simulink model "IDEAL_Diagrama_completo_prolijo"  (R2023b)
settings: Solver=VariableStepAuto  StartTime=0.0  StopTime=15  FixedStep=Ts  RelTol=1e-3
values from neighbouring files (symbols this model uses):
  A_corriente = [0 1; -wn_corriente^2 -2*zeta_corriente*wn_corriente]    [SensoresReales.m]
  A_inv = [0 1; -wn_inv^2 -2*zeta_inv*wn_inv]    [SensoresReales.m]
  A_temp = -1/tau_temp    (= -0.05)    [SensoresReales.m]
  A_tita = [0 1; -wn_tita^2 -2*zeta_tita*wn_tita]    [SensoresReales.m]
  B_corriente = [0; wn_corriente^2]    [SensoresReales.m]
  B_inv = [0; wn_inv^2]    [SensoresReales.m]
  B_temp = 1/tau_temp    (= 0.05)    [SensoresReales.m]
  B_tita = [0; wn_tita^2]    [SensoresReales.m]
  ba = Jeq * n * wn    [PolosPID.m]
  C_corriente = [1 0]    [SensoresReales.m]
  C_inv = [1 0]    [SensoresReales.m]
  C_temp = 1    [SensoresReales.m]
  C_tita = [1 0]    [SensoresReales.m]
  D_corriente = 0    [SensoresReales.m]
  D_inv = 0    [SensoresReales.m]
  D_temp = 0    [SensoresReales.m]
  D_tita = 0    [SensoresReales.m]
  ketita = double(sol.ketita_s)    [PIDPolosObsReducidoEst.m]    (also in PolosObsReducidoEst.m)
  kew = double(sol.kew_s)    [PIDPolosObsReducidoEst.m]    (also in PolosObsReducidoEst.m)
  kewint = double(sol.kewint_s)    [PIDPolosObsReducidoEst.m]    (also in PolosObsReducidoEst.m = 0)
  Ksa = Jeq * n * wn^2    [PolosPID.m]
  Ksia = Jeq * wn^3    [PolosPID.m]
  Ra_prima = Lq/Tau    [RaLazoControlCorriente.m]
  Tau = -1/Pi    (= 0.0002)    [RaLazoControlCorriente.m]
  Ts = 0.0001    [TustinPID.m]
undefined symbols (not defined in the file or in its folder): alfa, beq, Cts, dGi, dGsc, dGsp, dGsT, femax, g, gcbh, id0, io0, iq0, Ismax, Isnom, Jeq, KEeq, kl, KTeq, lambda_m, Ld, Lls, Lq, nGi, nGsc, nGsp, nGsT, Pp, r, Rs, Rts_amb, sps, sps_rtmsupport, tita0, Tqnom, Ts0, Tsmax, Vflnom, Vsat, Wlnom, wm0, Wmnom
libraries: simulink_extras x8, eeTransforms x4, simulink x4, SignalEditorBlockLib x3, spsPositiveSequencePLLDrivenLib x1, spsSecondOrderFilterLib x1, spsMeanVariableFrequencyLib x1, spsabctodq0Lib x1
settings Model: Creator=Julian  LastModifiedBy=Gustavo

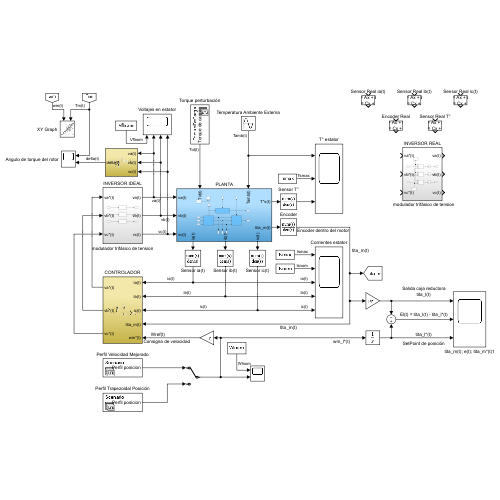
[thumbnail: Simulink's stored preview of the top-level diagram]
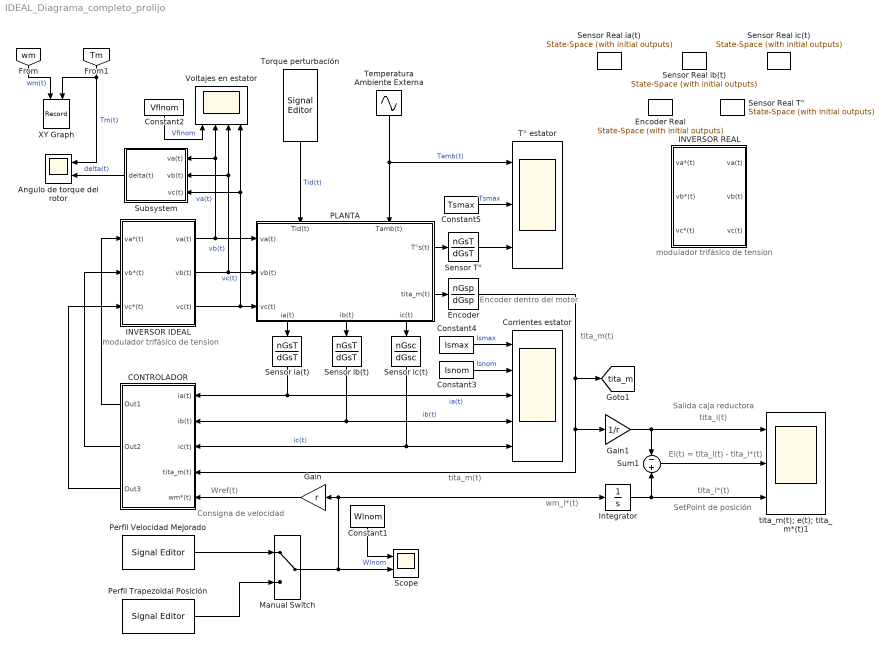
== system IDEAL_Diagrama_completo_prolijo ==
  note: modulador trifásico de tension
  note: SetPoint de posición
  note: Wref(t)
  note: Salida caja reductora
  note: Encoder dentro del motor
  note: tita_m(t)
  note: El(t) = tita_l(t) - tita_l*(t)
  note: tita_l*(t)
  note: tita_m(t)
  note: wm_l*(t)
  note: tita_l(t)
  note: Consigna de velocidad
  note: modulador trifásico de tension
  Angulo de torque del rotor : Scope  NumInputPorts=2
  CONTROLADOR : Subsystem
  Constant1 : Constant  Value=Wlnom
  Constant2 : Constant  Value=Vflnom
  Constant3 : Constant  Value=Isnom
  Constant4 : Constant  Value=Ismax
  Constant5 : Constant  Value=Tsmax
  Corrientes estator : Scope  NumInputPorts=5
  Encoder : TransferFcn  Numerator=nGsp  Denominator=dGsp
  Encoder Real : simulink_extras/Additional Linear/State-Space (with initial outputs)  A=A_tita  B=B_tita  C=C_tita  D=D_tita  U0=0  Y0=0
  Gain : Gain  Gain=r
  Gain1 : Gain  Gain=1/r
  INVERSOR IDEAL : Subsystem
  INVERSOR REAL : Subsystem
  Integrator : Integrator
  Manual Switch : ManualSwitch
  PLANTA : Subsystem
      settings: PortSchema="{\"entries\":[{\"content\":{\"sides\":[{\"content\":{\"connectorIds\":[\"In1\",\"In2\",\"In3\"]},\"type\":\"ConnectorPlacement.EquallySpacedRectSide\",\"uuid\":\"c9ff8e03-575d-49b6-9d53-263c6173ec7a\"},{\"content\":{\"connectorIds\":[\"Out1\",\"Out2\"],\"side\":\"RIGHT\"},\"type\":\"ConnectorPlacement.EquallySpacedRectSide\",\"uuid\":\"b812656a-111e-4032-91bd-eba1e3276cdf\"},{\"content\":{\"connectorIds\":[\"In4\",\"In5\"],\"side\":\"TOP\"},\"type\":\"ConnectorPlacement.EquallySpacedRectSide\",\"uuid\":\"1a03caaa-7f6e-4ad3-ab54-ee47607f786a\"},{\"content\":{\"connectorIds\":[\"Out3\",\"Out4\",\"Out5\"],\"side\":\"BOTTOM\"},\"type\":\"ConnectorPlacement.EquallySpacedRectSide\",\"uuid\":\"9d23a867-d392-4f38-a76b-2655c4618fc4\"}]},\"type\":\"ConnectorPlacement.EquallySpacedConnector\",\"uuid\":\"9323b1ce-1fa4-461e-b8aa-3e94b35b1dab\"}],\"packageUris\":[\"http://schema.mathworks.com/mf0/Connector/R2020b\"],\"version\":\"1.0\"}"
  Perfil Trapezoidal Posición : SignalEditorBlockLib/Signal Editor  FileName=Perfil trapezoidal de posicion.mat  ActiveScenario=Scenario  ActiveSignal=Perfil posicion  IsBus=off  OutputBusObjectStr=Bus: BusObject  SampleTime=0  ZeroCross=off  OutputAfterFinalValue=Setting to zero  Unit=inherit  PreserveSignalName=on  ApplySigPropsToAllScenarios=on  ApplySigPropsToAllSignals=off
  Perfil Velocidad Mejorado : SignalEditorBlockLib/Signal Editor  FileName=PerfilTrapezoidalVelocidadMejorado.mat  ActiveScenario=Scenario  ActiveSignal=Perfil posicion  IsBus=off  OutputBusObjectStr=Bus: BusObject  SampleTime=0  ZeroCross=off  OutputAfterFinalValue=Setting to zero  Unit=inherit  PreserveSignalName=on  ApplySigPropsToAllScenarios=on  ApplySigPropsToAllSignals=off
  Scope : Scope  NumInputPorts=2
  Sensor Real T° : simulink_extras/Additional Linear/State-Space (with initial outputs)  A=A_temp  B=B_temp  C=C_temp  D=D_temp  U0=Ts0  Y0=Ts0
  Sensor Real ia(t) : simulink_extras/Additional Linear/State-Space (with initial outputs)  A=A_corriente  B=B_corriente  C=C_corriente  D=D_corriente  U0=0  Y0=0
  Sensor Real ib(t) : simulink_extras/Additional Linear/State-Space (with initial outputs)  A=A_corriente  B=B_corriente  C=C_corriente  D=D_corriente  U0=0  Y0=0
  Sensor Real ic(t) : simulink_extras/Additional Linear/State-Space (with initial outputs)  A=A_corriente  B=B_corriente  C=C_corriente  D=D_corriente  U0=0  Y0=0
  Sensor T° : TransferFcn  Numerator=nGsT  Denominator=dGsT
  Sensor ia(t) : TransferFcn  Numerator=nGsT  Denominator=dGsT
  Sensor ib(t) : TransferFcn  Numerator=nGsT  Denominator=dGsT
  Sensor ic(t) : TransferFcn  Numerator=nGsc  Denominator=dGsc
  Subsystem : Subsystem
  Sum1 : Sum  Inputs=-|+
  Temperatura Ambiente Externa : Sin  Amplitude=27.5  Bias=12.5  Frequency=2*pi/15  Phase=pi/2  SampleTime=0
  Torque perturbación : SignalEditorBlockLib/Signal Editor  FileName=Torque de carga Tdl(t).mat  ActiveScenario=TorqueDeCarga  ActiveSignal=Torque de carga  IsBus=off  OutputBusObjectStr=Bus: BusObject  SampleTime=0  ZeroCross=off  OutputAfterFinalValue=Setting to zero  Unit=N*m  PreserveSignalName=on  ApplySigPropsToAllScenarios=on  ApplySigPropsToAllSignals=off
  T° estator : Scope  NumInputPorts=3
  Voltajes en estator : Scope  NumInputPorts=4
  XY Graph : Record  FileSettingsInternal="{\"entries\":[{\"content\":{\"excelSettings\":{\"content\":{},\"type\":\"Streamout.ExcelSettings\"}},\"type\":\"Streamout.FileSettingStorage\",\"uuid\":\"\"}],\"packageUris\":[\"http:\\/\\/schema.mathworks.com\\/mf0\\/streamout_blocks\\/R2020a\"],\"version\":\"1.0\"}"  Layout=[1 1]  SignalsInternal="{\"entries\":[{\"content\":{\"signals\":[{\"content\":{\"blockPath\":[],\"dimensions\":[1],\"domain\":\"\",\"lineColor\":\"#a2142f\",\"plots\":[1],\"port\":1,\"sid\":[\"\"],\"signalID\":587,\"signalName\":\"wm(t)\"},\"type\":\"RecordBlkView.Signal\",\"uuid\":\"\"},{\"content\":{\"blockPath\":[],\"dimensions\":[1],\"domain\":\"\",\"lineColor\":\"#139fff\",\"plots\":[1],\"port\":2,\"sid\":[\"\"],\"signalID\":591,\"signalName\":\"Tm(t)\"},\"type\":\"RecordBlkView.Signal\",\"uuid\":\"\"}]},\"type\":\"RecordBlkView.InputSignals\",\"uuid\":\"\"}],\"packageUris\":[\"http:\\/\\/schema.mathworks.com\\/mf0\\/streamout_blocks\\/R2020a\"],\"version\":\"1.0\"}"  VisualizationBindings="{\"xyplotplugin\":{\"info\":[{\"series\":[{\"bindingParametersList\":[{\"parameter\":\"Y-Axis\",\"signalID\":591,\"signalName\":\"Tm(t)\"},{\"parameter\":\"X-Axis\",\"signalID\":587,\"signalName\":\"wm(t)\"}],\"seriesID\":55069}],\"subplotID\":1}]}}"  CompatibilityTag=XY
  tita_m(t); e(t); tita_m*(t)1 : Scope  NumInputPorts=3
  tag scope: tita_m=global
  wires:
  INVERSOR IDEAL/1(va(t)) -> PLANTA/1(va(t)), Voltajes en estator/2, Subsystem/1(va(t))  "va(t)"
  INVERSOR IDEAL/2(vb(t)) -> PLANTA/2(vb(t)), Voltajes en estator/3, Subsystem/2(vb(t))  "vb(t)"
  INVERSOR IDEAL/3(vc(t)) -> Voltajes en estator/4, Subsystem/3(vc(t)), PLANTA/3(vc(t))  "vc(t)"
  CONTROLADOR/1(Out1) -> INVERSOR IDEAL/1(va*(t))
  CONTROLADOR/2(Out2) -> INVERSOR IDEAL/2(vb*(t))
  CONTROLADOR/3(Out3) -> INVERSOR IDEAL/3(vc*(t))
  Sensor T°/1 -> T° estator/3
  Gain/1 -> CONTROLADOR/5(wm*(t))
  Encoder/1 -> CONTROLADOR/4(tita_m(t)), Gain1/1, [tita_m]
  Gain1/1 -> tita_m(t); e(t); tita_m*(t)1/1, Sum1/1
  Sum1/1 -> tita_m(t); e(t); tita_m*(t)1/2
  Integrator/1 -> Sum1/2, tita_m(t); e(t); tita_m*(t)1/3
  PLANTA/3(ia(t)) -> Sensor ia(t)/1
  PLANTA/4(ib(t)) -> Sensor ib(t)/1
  PLANTA/5(ic(t)) -> Sensor ic(t)/1
  Temperatura Ambiente Externa/1 -> PLANTA/5(Tamb(t)), T° estator/1  "Tamb(t)"
  Torque perturbación/1 -> PLANTA/4(Tid(t))  "Tid(t)"
  PLANTA/2(tita_m(t)) -> Encoder/1
  PLANTA/1(T°s(t)) -> Sensor T°/1
  Sensor ic(t)/1 -> CONTROLADOR/3(ic(t)), Corrientes estator/5  "ic(t)"
  Sensor ib(t)/1 -> CONTROLADOR/2(ib(t)), Corrientes estator/4  "ib(t)"
  Sensor ia(t)/1 -> CONTROLADOR/1(ia(t)), Corrientes estator/3  "ia(t)"
  Manual Switch/1 -> Scope/2, Integrator/1, Gain/1
  Perfil Trapezoidal Posición/1 -> Manual Switch/2
  Perfil Velocidad Mejorado/1 -> Manual Switch/1
  Constant1/1 -> Scope/1  "Wlnom"
  Constant2/1 -> Voltajes en estator/1  "Vflnom"
  Constant3/1 -> Corrientes estator/2  "Isnom"
  Constant4/1 -> Corrientes estator/1  "Ismax"
  Subsystem/1(delta(t)) -> Angulo de torque del rotor/2  "delta(t)"
  [Tm] -> Angulo de torque del rotor/1, XY Graph/2  "Tm(t)"
  [wm] -> XY Graph/1  "wm(t)"
  Constant5/1 -> T° estator/2  "Tsmax"

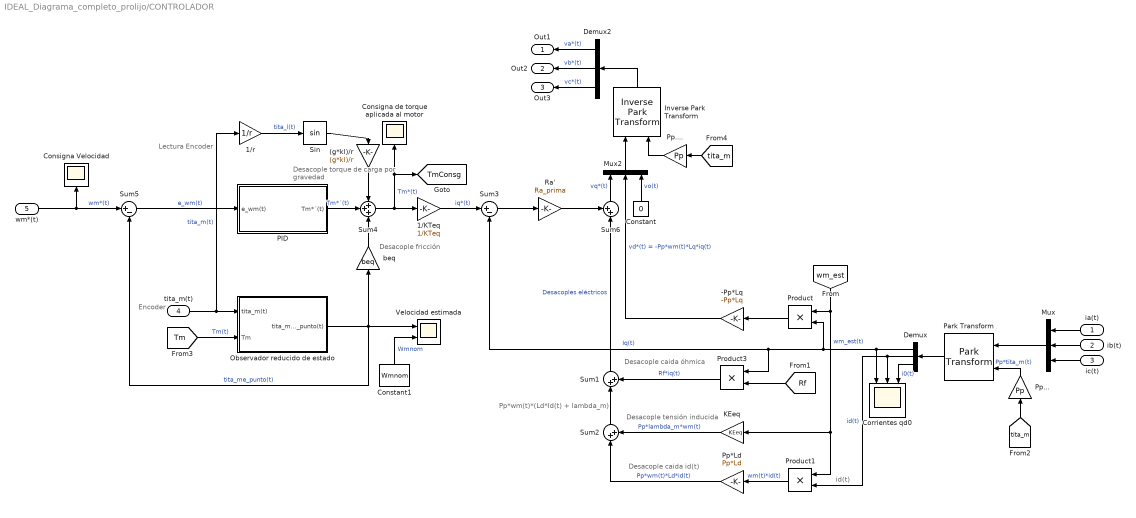
== system IDEAL_Diagrama_completo_prolijo/CONTROLADOR ==
  note: id(t)
  note: Desacople caida id(t)
  note: Encoder
  note: Desacople caida óhmica
  note: Desacople fricción
  note: Desacople tensión inducida
  note: Pp*wm(t)*(Ld*Id(t) + lambda_m)
  note: Lectura Encoder
  note: Desacople torque
      | de carga por gravedad
  ia(t) : Inport
  ib(t) : Inport  Port=2
  ic(t) : Inport  Port=3
  tita_m(t) : Inport  Port=4
  wm*(t) : Inport  Port=5
  (g*kl)/r : Gain  Gain=(g*kl)/r
  -Pp*Lq : Gain  Gain=-Pp*Lq
  1/KTeq : Gain  Gain=1/KTeq
  1/r : Gain  Gain=1/r
  Consigna Velocidad : Scope
  Consigna de torque aplicada al motor : Scope
  Constant : Constant  Value=0
  Constant1 : Constant  Value=Wmnom
  Corrientes qd0 : Scope  NumInputPorts=3
  Demux : Demux  Outputs=3
  Demux2 : Demux  Outputs=3
  Inverse Park Transform : eeTransforms/Inverse Park Transform  AxisAlignment=Q-axis  PowerInvariant=off
      settings: LibrarySourceBlock=|
      | ee_sl_lib/Mathematical
      | Transforms/Inverse
      | Park Transform
  KEeq : Gain  Gain=KEeq
  Mux : Mux  Inputs=3
  Mux2 : Mux  Inputs=3
  Observador reducido de estado : Subsystem
  PID : Subsystem
  Park Transform : eeTransforms/Park Transform  AxisAlignment=Q-axis  PowerInvariant=off
      settings: LibrarySourceBlock=|
      | ee_sl_lib/Mathematical
      | Transforms/Park Transform
  Pp*Ld : Gain  Gain=Pp*Ld
  Pp... : Gain  Gain=Pp
  Pp.... : Gain  Gain=Pp
  Product : Product
  Product1 : Product
  Product3 : Product
  Ra' : Gain  Gain=Ra_prima
  Sin : Trigonometry
  Sum1 : Sum  Inputs=|++
  Sum2 : Sum  Inputs=|++
  Sum3 : Sum  Inputs=|+-
  Sum4 : Sum  Inputs=+++
  Sum5 : Sum  Inputs=|+-
  Sum6 : Sum  Inputs=++|
  Velocidad estimada : Scope  NumInputPorts=2
  beq : Gain  Gain=beq
  Out1 : Outport
  Out2 : Outport  Port=2
  Out3 : Outport  Port=3
  tag scope: TmConsg=global
  wires:
  Mux/1 -> Park Transform/1
  [tita_m] -> Pp..../1
  Pp..../1 -> Inverse Park Transform/2
  Demux2/2 -> Out2/1  "vb*(t)"
  Sum3/1 -> Ra'/1
  Constant/1 -> Mux2/3  "vo(t)"
  Demux2/1 -> Out1/1  "va*(t)"
  -Pp*Lq/1 -> Mux2/2  "vd*(t) = -Pp*wm(t)*Lq*iq(t)"
  Product3/1 -> Sum1/2  "Rf*iq(t)"
  [tita_m] -> Pp.../1
  Ra'/1 -> Sum6/1
  Inverse Park Transform/1 -> Demux2/1
  KEeq/1 -> Sum2/2  "Pp*lambda_m*wm(t)"
  Product1/1 -> Pp*Ld/1  "wm(t)*id(t)"
  Mux2/1 -> Inverse Park Transform/1
  Sum2/1 -> Sum1/1
  wm*(t)/1 -> Sum5/1, Consigna Velocidad/1  "wm*(t)"
  Pp*Ld/1 -> Sum2/1  "Pp*wm(t)*Ld*id(t)"
  1/KTeq/1 -> Sum3/1  "iq*(t)"
  Product/1 -> -Pp*Lq/1
  ia(t)/1 -> Mux/1
  Park Transform/1 -> Demux/1
  Pp.../1 -> Park Transform/2  "Pp*tita_m(t)"
  Sum6/1 -> Mux2/1  "vq*(t)"
  Demux2/3 -> Out3/1  "vc*(t)"
  ib(t)/1 -> Mux/2
  tita_m(t)/1 -> 1/r/1, Observador reducido de estado/1(tita_m(t))  "tita_m(t)"
  [Tm] -> Observador reducido de estado/2(Tm)  "Tm(t)"
  [Rf] -> Product3/2
  ic(t)/1 -> Mux/3
  Sum5/1 -> PID/1(e_wm(t))  "e_wm(t)"
  Sum1/1 -> Sum6/2  "Desacoples eléctricos"
  PID/1(Tm*´(t)) -> Sum4/2  "Tm*´(t)"
  Sum4/1 -> 1/KTeq/1, Consigna de torque aplicada al motor/1, [TmConsg]  "Tm*(t)"
  beq/1 -> Sum4/3
  Observador reducido de estado/1(tita_me_punto(t)) -> beq/1, Velocidad estimada/1, Sum5/2  "tita_me_punto(t)"
  Demux/3 -> Corrientes qd0/3  "i0(t)"
  Demux/2 -> Product1/2, Corrientes qd0/2  "id(t)"
  Demux/1 -> Product3/1, Sum3/2, Product/2, Corrientes qd0/1  "Iq(t)"
  1/r/1 -> Sin/1  "tita_l(t)"
  Sin/1 -> (g*kl)/r/1
  (g*kl)/r/1 -> Sum4/1
  [wm_est] -> Product/1, Product1/1, KEeq/1  "wm_est(t)"
  Constant1/1 -> Velocidad estimada/2  "Wmnom"

== system IDEAL_Diagrama_completo_prolijo/INVERSOR IDEAL ==
  va*(t) : Inport
  vb*(t) : Inport  Port=2
  vc*(t) : Inport  Port=3
  Inversor fase a : TransferFcn  Numerator=nGi  Denominator=dGi
  Inversor fase b : TransferFcn  Numerator=nGi  Denominator=dGi
  Inversor fase c : TransferFcn  Numerator=nGi  Denominator=dGi
  va(t) : Outport
  vb(t) : Outport  Port=2
  vc(t) : Outport  Port=3
  wires:
  Inversor fase c/1 -> vc(t)/1  "vc(t)"
  va*(t)/1 -> Inversor fase a/1
  Inversor fase a/1 -> va(t)/1  "va(t)"
  vc*(t)/1 -> Inversor fase c/1
  Inversor fase b/1 -> vb(t)/1  "vb(t)"
  vb*(t)/1 -> Inversor fase b/1

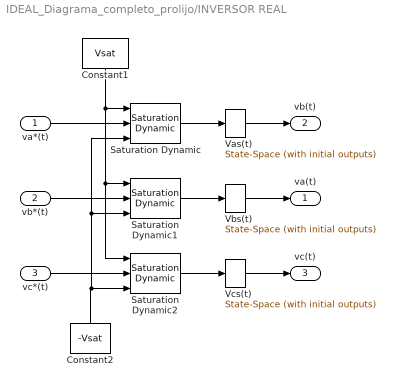
== system IDEAL_Diagrama_completo_prolijo/INVERSOR REAL ==
  va*(t) : Inport
  vb*(t) : Inport  Port=2
  vc*(t) : Inport  Port=3
  Constant1 : Constant  Value=Vsat
  Constant2 : Constant  Value=-Vsat
  Saturation Dynamic : simulink/Discontinuities/Saturation Dynamic  OutMin=[]  OutMax=[]  OutDataTypeStr=Inherit: Same as second input  OutDataType=fixdt(1, 16)  OutScaling=2^-10  DoSatur=off
  Saturation Dynamic1 : simulink/Discontinuities/Saturation Dynamic  OutMin=[]  OutMax=[]  OutDataTypeStr=Inherit: Same as second input  OutDataType=fixdt(1, 16)  OutScaling=2^-10  DoSatur=off
  Saturation Dynamic2 : simulink/Discontinuities/Saturation Dynamic  OutMin=[]  OutMax=[]  OutDataTypeStr=Inherit: Same as second input  OutDataType=fixdt(1, 16)  OutScaling=2^-10  DoSatur=off
  "Vas(t) " : simulink_extras/Additional Linear/State-Space (with initial outputs)  A=A_inv  B=B_inv  C=C_inv  D=D_inv  U0=0  Y0=0
  "Vbs(t) " : simulink_extras/Additional Linear/State-Space (with initial outputs)  A=A_inv  B=B_inv  C=C_inv  D=D_inv  U0=0  Y0=0
  "Vcs(t) " : simulink_extras/Additional Linear/State-Space (with initial outputs)  A=A_inv  B=B_inv  C=C_inv  D=D_inv  U0=0  Y0=0
  va(t) : Outport
  vb(t) : Outport  Port=2
  vc(t) : Outport  Port=3
  wires:
  va*(t)/1 -> Saturation Dynamic/2
  vb*(t)/1 -> Saturation Dynamic1/2
  vc*(t)/1 -> Saturation Dynamic2/2
  Constant2/1 -> Saturation Dynamic2/3, Saturation Dynamic/3, Saturation Dynamic1/3
  Saturation Dynamic/1 -> "Vas(t) "/1
  "Vas(t) "/1 -> vb(t)/1
  Saturation Dynamic1/1 -> "Vbs(t) "/1
  Saturation Dynamic2/1 -> "Vcs(t) "/1
  "Vbs(t) "/1 -> va(t)/1
  "Vcs(t) "/1 -> vc(t)/1
  Constant1/1 -> Saturation Dynamic2/1, Saturation Dynamic1/1, Saturation Dynamic/1

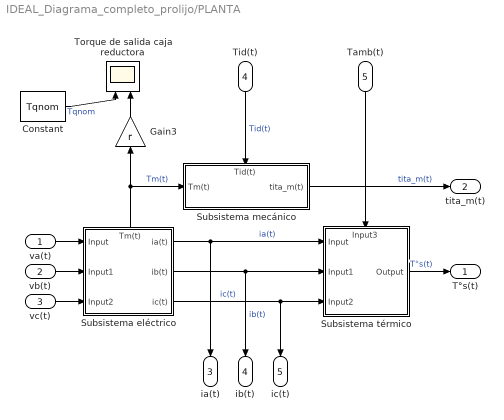
== system IDEAL_Diagrama_completo_prolijo/PLANTA ==
  va(t) : Inport
  vb(t) : Inport  Port=2
  vc(t) : Inport  Port=3
  Tid(t) : Inport  Port=4
  Tamb(t) : Inport  Port=5
  Constant : Constant  Value=Tqnom
  Gain3 : Gain  Gain=r
  Subsistema eléctrico : Subsystem
      settings: PortSchema="{\"entries\":[{\"content\":{\"sides\":[{\"content\":{\"connectorIds\":[\"In1\",\"In2\",\"In3\"]},\"type\":\"ConnectorPlacement.EquallySpacedRectSide\",\"uuid\":\"55314de5-b6ab-4161-b15d-819ac9b3d610\"},{\"content\":{\"connectorIds\":[\"Out1\",\"Out2\",\"Out3\"],\"side\":\"RIGHT\"},\"type\":\"ConnectorPlacement.EquallySpacedRectSide\",\"uuid\":\"6d89c228-26ff-4db5-b942-5bfef0be2fde\"},{\"content\":{\"connectorIds\":[\"Out4\"],\"side\":\"TOP\"},\"type\":\"ConnectorPlacement.EquallySpacedRectSide\",\"uuid\":\"a52f3ca3-a7f6-4886-b92b-9c9e6a107711\"}]},\"type\":\"ConnectorPlacement.EquallySpacedConnector\",\"uuid\":\"22991da4-d60d-4ddc-8bfe-b68e23663f11\"}],\"packageUris\":[\"http://schema.mathworks.com/mf0/Connector/R2020b\"],\"version\":\"1.0\"}"
  Subsistema mecánico : Subsystem
      settings: PortSchema="{\"entries\":[{\"content\":{\"sides\":[{\"content\":{\"connectorIds\":[\"In1\"]},\"type\":\"ConnectorPlacement.EquallySpacedRectSide\",\"uuid\":\"db0c31ff-fb9a-4cce-bd75-6b297d65744d\"},{\"content\":{\"connectorIds\":[\"Out1\"],\"side\":\"RIGHT\"},\"type\":\"ConnectorPlacement.EquallySpacedRectSide\",\"uuid\":\"ab44173d-bb84-4ea2-b7b7-ef15b1ff9d5e\"},{\"content\":{\"connectorIds\":[\"In2\"],\"side\":\"TOP\"},\"type\":\"ConnectorPlacement.EquallySpacedRectSide\",\"uuid\":\"a2ba5669-abba-4e87-b14b-37ec0d904023\"}]},\"type\":\"ConnectorPlacement.EquallySpacedConnector\",\"uuid\":\"7722c9ef-afaa-4930-9e2a-97c0dfb446ab\"}],\"packageUris\":[\"http://schema.mathworks.com/mf0/Connector/R2020b\"],\"version\":\"1.0\"}"
  Subsistema térmico : Subsystem
      settings: PortSchema="{\"entries\":[{\"content\":{\"sides\":[{\"content\":{\"connectorIds\":[\"In1\",\"In2\",\"In3\"]},\"type\":\"ConnectorPlacement.EquallySpacedRectSide\",\"uuid\":\"499bb5e3-da94-498d-be5e-1974ba0b4a58\"},{\"content\":{\"connectorIds\":[\"Out1\"],\"side\":\"RIGHT\"},\"type\":\"ConnectorPlacement.EquallySpacedRectSide\",\"uuid\":\"13ea5dea-e51e-4770-b579-88e3e6e50884\"},{\"content\":{\"connectorIds\":[\"In4\"],\"side\":\"TOP\"},\"type\":\"ConnectorPlacement.EquallySpacedRectSide\",\"uuid\":\"72517ed1-a98f-428e-86e2-c370e237c602\"}]},\"type\":\"ConnectorPlacement.EquallySpacedConnector\",\"uuid\":\"7e0eda24-12d6-49d0-ad1f-024c88e78140\"}],\"packageUris\":[\"http://schema.mathworks.com/mf0/Connector/R2020b\"],\"version\":\"1.0\"}"
  Torque de salida caja reductora : Scope  NumInputPorts=2
  T°s(t) : Outport
  tita_m(t) : Outport  Port=2
  ia(t) : Outport  Port=3
  ib(t) : Outport  Port=4
  ic(t) : Outport  Port=5
  wires:
  Tamb(t)/1 -> Subsistema térmico/4(Input3)
  Subsistema eléctrico/3(ic(t)) -> Subsistema térmico/3(Input2), ic(t)/1  "ic(t)"
  Subsistema eléctrico/1(ia(t)) -> Subsistema térmico/1(Input), ia(t)/1  "ia(t)"
  Subsistema térmico/1(Output) -> T°s(t)/1  "T°s(t)"
  Subsistema eléctrico/4(Tm(t)) -> Gain3/1, Subsistema mecánico/1(Tm(t))  "Tm(t)"
  Subsistema eléctrico/2(ib(t)) -> Subsistema térmico/2(Input1), ib(t)/1  "ib(t)"
  Subsistema mecánico/1(tita_m(t)) -> tita_m(t)/1  "tita_m(t)"
  va(t)/1 -> Subsistema eléctrico/1(Input)
  vb(t)/1 -> Subsistema eléctrico/2(Input1)
  Tid(t)/1 -> Subsistema mecánico/2(Tid(t))  "Tid(t)"
  vc(t)/1 -> Subsistema eléctrico/3(Input2)
  Gain3/1 -> Torque de salida caja reductora/2
  Constant/1 -> Torque de salida caja reductora/1  "Tqnom"

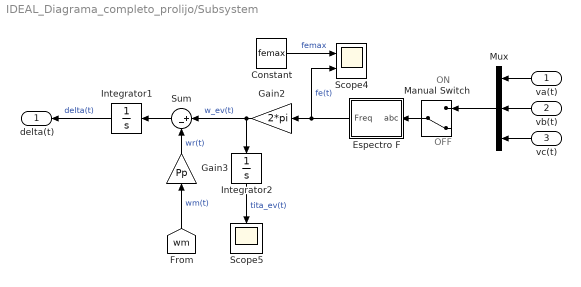
== system IDEAL_Diagrama_completo_prolijo/Subsystem ==
  note: OFF
  note: ON
  va(t) : Inport
  vb(t) : Inport  Port=2
  vc(t) : Inport  Port=3
  Constant : Constant  Value=femax
  Espectro F : Subsystem  AncestorBlock=|  DialogController=POWERSYS.PowerSysDialog  LoadFcn=sps_rtmsupport('LoadFcn', gcbh);  StartFcn=sps_rtmsupport('StartFcn', gcbh);  StopFcn=sps_rtmsupport('StopFcn', gcbh);  mask(PLL (3ph)){Fmin=45, Par_Init=[0, 50], ParK=[180, 3200, 1], TcD=1e-4, MaxRateChangeFreq=12, FilterCutOffFreq=25, Ts=0, AGC=on}
      | sps_lib/Control/PLL
      | (3ph)
      mask prompts: Fmin "Minimum frequency (Hz):"; Par_Init "Initial inputs [ Phase (degrees), Frequency (Hz) ]:"; ParK "Regulator gains [ Kp, Ki, Kd ]:"; TcD "Time constant for derivative action (s):"; MaxRateChangeFreq "Maximum rate of change of frequency (Hz/s):"; FilterCutOffFreq "Filter cut-off frequency for frequency measurement (Hz):"; Ts "Sample time:"; AGC "Enable automatic gain control"
      mask help:
      | This Phase Locked Loop (PLL) system can be used  to synchronize on a set of variable frequency, three-phase sinusoidal signals. If the Automatic Gain Control is enabled, the input (phase error) of the PLL regulator is scaled according to the input signals magnitude.
      |
      | For optimal performance, set regulator gains [ Kp Ki  Kd ] = [ 180  3200  1 ] and check the Enable Automatic Gain Control parameter.
      |
      | Input : Vector containing the normalized three-phase signals [Va Vb Vc]
      | Output 1:  Measured frequency (Hz) = w/(2pi)
      | Output 2:  Ramp w.t varying between  0 and 2*pi, synchronized on zero crossings of the fundamental (positive-sequence) of phase A.
      mask init:
      | block=gcb;
      | [WantBlockChoice,Ts,sps] = powericon('PLL3phInit',block,Fmin,Par_Init,ParK,TcD, MaxRateChangeFreq, FilterCutOffFreq, AGC,Ts);
      | powericon('SetInternalModels','set',block,WantBlockChoice);
      settings: CopyFcn=sps_rtmsupport('CopyFcn', gcbh);  DeleteFcn=sps_rtmsupport('DeleteFcn', gcbh);  UndoDeleteFcn=sps_rtmsupport('UndoDeleteFcn', gcbh);  ModelCloseFcn=sps_rtmsupport('ModelCloseFcn', gcbh);  PreSaveFcn=sps_rtmsupport('PreSaveFcn', gcbh);  PostSaveFcn=sps_rtmsupport('PostSaveFcn', gcbh);  NameChangeFcn=sps_rtmsupport('NameChangeFcn', gcbh);  PreCopyFcn=sps_rtmsupport('PreCopyFcn', gcbh);  OpenFcn=sps_rtmsupport('OpenFcn', gcbh, [8]);  CloseFcn=sps_rtmsupport('CloseFcn', gcbh);  PreDeleteFcn=sps_rtmsupport('PreDeleteFcn', gcbh);
      settings: LibrarySourceBlock=|
      | sps_lib/Control/PLL
      | (3ph)
      mask Help: helpview(psbhelp);
  Gain2 : Gain  Gain=2*pi
  Gain3 : Gain  Gain=Pp
  Integrator1 : Integrator
  Integrator2 : Integrator
  Manual Switch : ManualSwitch  CurrentSetting=0
  Mux : Mux  Inputs=3
  Scope4 : Scope  NumInputPorts=2
  Scope5 : Scope
  Sum : Sum  Inputs=|+-
  delta(t) : Outport
  wires:
  Gain3/1 -> Sum/2  "wr(t)"
  Constant/1 -> Scope4/1  "femax"
  Sum/1 -> Integrator1/1
  Espectro F/1(Freq) -> Gain2/1, Scope4/2  "fe(t)"
  vb(t)/1 -> Mux/2
  Gain2/1 -> Sum/1, Integrator2/1  "w_ev(t)"
  Integrator2/1 -> Scope5/1  "tita_ev(t)"
  [wm] -> Gain3/1  "wm(t)"
  vc(t)/1 -> Mux/3
  va(t)/1 -> Mux/1
  Integrator1/1 -> delta(t)/1  "delta(t)"
  Mux/1 -> Manual Switch/1
  Manual Switch/1 -> Espectro F/1(abc)

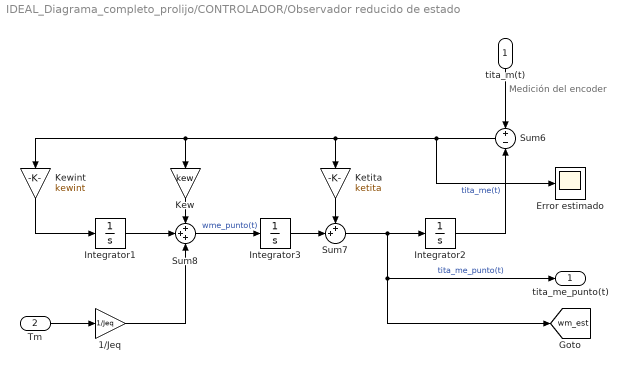
== system IDEAL_Diagrama_completo_prolijo/CONTROLADOR/Observador reducido de estado ==
  note: Medición del encoder
  tita_m(t) : Inport
  Tm : Inport  Port=2
  1/Jeq : Gain  Gain=1/Jeq
  Error estimado : Scope
  Integrator1 : Integrator
  Integrator2 : Integrator
  Integrator3 : Integrator
  Ketita : Gain  Gain=ketita
  Kew : Gain  Gain=kew
  Kewint : Gain  Gain=kewint
  Sum6 : Sum  Inputs=+-
  Sum7 : Sum  Inputs=++|
  Sum8 : Sum  Inputs=+++
  tita_me_punto(t) : Outport
  tag scope: wm_est=global
  wires:
  Sum7/1 -> [wm_est], tita_me_punto(t)/1, Integrator2/1  "tita_me_punto(t)"
  Sum6/1 -> Error estimado/1, Kewint/1, Kew/1, Ketita/1
  Integrator3/1 -> Sum7/2
  Integrator2/1 -> Sum6/2  "tita_me(t)"
  Kew/1 -> Sum8/1
  Ketita/1 -> Sum7/1
  Sum8/1 -> Integrator3/1  "wme_punto(t)"
  tita_m(t)/1 -> Sum6/1
  Tm/1 -> 1/Jeq/1
  1/Jeq/1 -> Sum8/3
  Kewint/1 -> Integrator1/1
  Integrator1/1 -> Sum8/2

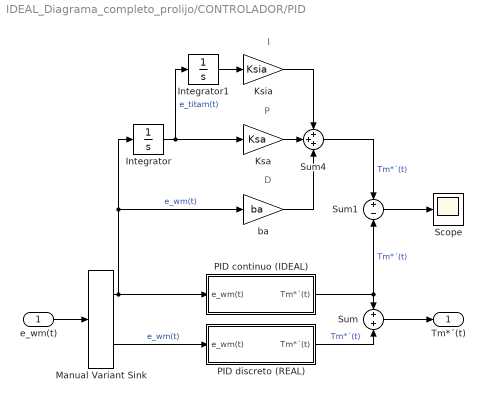
== system IDEAL_Diagrama_completo_prolijo/CONTROLADOR/PID ==
  note: I
  note: D
  note: P
  e_wm(t) : Inport
  Integrator : Integrator
  Integrator1 : Integrator
  Ksa : Gain  Gain=Ksa
  Ksia : Gain  Gain=Ksia
  Manual Variant Sink : simulink/Signal Routing/Manual Variant Sink  NumChoices=2  LabelModeActiveChoice=V_1
  PID continuo (IDEAL) : Subsystem
  PID discreto (REAL) : Subsystem
  Scope : Scope
  Sum : Sum  Inputs=+|+
  Sum1 : Sum  Inputs=+|-
  Sum4 : Sum  Inputs=+++
  ba : Gain  Gain=ba
  Tm*´(t) : Outport
  wires:
  Sum4/1 -> Sum1/1  "Tm*´(t)"
  Ksa/1 -> Sum4/2
  Ksia/1 -> Sum4/1
  Integrator/1 -> Integrator1/1, Ksa/1  "e_titam(t)"
  ba/1 -> Sum4/3
  Integrator1/1 -> Ksia/1
  e_wm(t)/1 -> Manual Variant Sink/1
  Manual Variant Sink/1 -> PID continuo (IDEAL)/1(e_wm(t)), ba/1, Integrator/1  "e_wm(t)"
  Manual Variant Sink/2 -> PID discreto (REAL)/1(e_wm(t))  "e_wm(t)"
  PID discreto (REAL)/1(Tm*´(t)) -> Sum/2  "Tm*´(t)"
  PID continuo (IDEAL)/1(Tm*´(t)) -> Sum1/2, Sum/1  "Tm*´(t)"
  Sum1/1 -> Scope/1
  Sum/1 -> Tm*´(t)/1

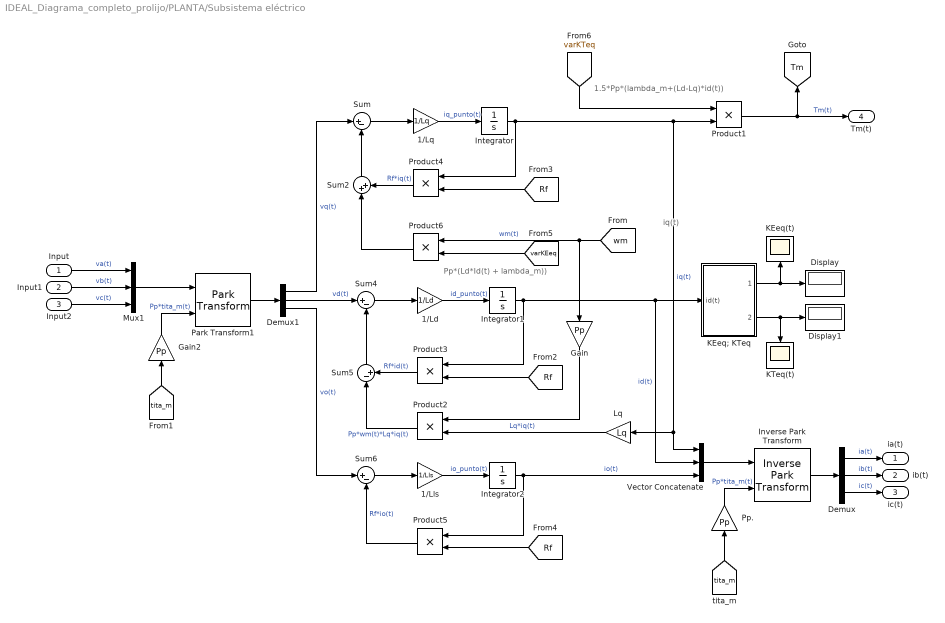
== system IDEAL_Diagrama_completo_prolijo/PLANTA/Subsistema eléctrico ==
  note: 1.5*Pp*(lambda_m+(Ld-Lq)*id(t))
  note: iq(t)
  note: Pp*(Ld*Id(t) + lambda_m))
  Input : Inport
  Input1 : Inport  Port=2
  Input2 : Inport  Port=3
  1/Ld : Gain  Gain=1/Ld
  1/Lls : Gain  Gain=1/Lls
  1/Lq : Gain  Gain=1/Lq
  Demux : Demux  Outputs=3
  Demux1 : Demux  Outputs=3
  Display : Display
  Display1 : Display
  Gain : Gain  Gain=Pp
  Gain2 : Gain  Gain=Pp
  Integrator : Integrator  InitialCondition=iq0
  Integrator1 : Integrator  InitialCondition=id0
  Integrator2 : Integrator  InitialCondition=io0
  Inverse Park Transform : eeTransforms/Inverse Park Transform  AxisAlignment=Q-axis  PowerInvariant=off
      settings: LibrarySourceBlock=|
      | ee_sl_lib/Mathematical
      | Transforms/Inverse
      | Park Transform
  KEeq(t) : Scope
  KEeq; KTeq : Subsystem
  KTeq(t) : Scope
  Lq : Gain  Gain=Lq
  Mux1 : Mux  Inputs=3
  Park Transform1 : eeTransforms/Park Transform  AxisAlignment=Q-axis  PowerInvariant=off
      settings: LibrarySourceBlock=|
      | ee_sl_lib/Mathematical
      | Transforms/Park Transform
  Pp. : Gain  Gain=Pp
  Product{1..6} (6 alike) : Product
  Sum : Sum  Inputs=|+-
  Sum2 : Sum  Inputs=|++
  Sum4 : Sum  Inputs=|+-
  Sum5 : Sum  Inputs=|-+
  Sum6 : Sum  Inputs=|+-
  Vector Concatenate : Concatenate  NumInputs=3
  ia(t) : Outport
  ib(t) : Outport  Port=2
  ic(t) : Outport  Port=3
  Tm(t) : Outport  Port=4
  tag scope: Tm=global
  wires:
  Sum4/1 -> 1/Ld/1
  Demux1/1 -> Sum/1  "vq(t)"
  Integrator/1 -> Product4/1, Product1/2, Lq/1, Vector Concatenate/1  "iq(t)"
  Product4/1 -> Sum2/2  "Rf*iq(t)"
  Pp./1 -> Inverse Park Transform/2  "Pp*tita_m(t)"
  Lq/1 -> Product2/2  "Lq*iq(t)"
  Sum/1 -> 1/Lq/1
  Sum2/1 -> Sum/2
  Demux1/3 -> Sum6/1  "vo(t)"
  Vector Concatenate/1 -> Inverse Park Transform/1
  1/Ld/1 -> Integrator1/1  "id_punto(t)"
  Inverse Park Transform/1 -> Demux/1
  1/Lls/1 -> Integrator2/1  "io_punto(t)"
  Sum5/1 -> Sum4/2
  Demux/3 -> ic(t)/1  "ic(t)"
  Demux/1 -> ia(t)/1  "ia(t)"
  Product3/1 -> Sum5/2  "Rf*id(t)"
  Demux/2 -> ib(t)/1  "ib(t)"
  Integrator2/1 -> Product5/1, Vector Concatenate/3  "io(t)"
  [tita_m] -> Pp./1
  Demux1/2 -> Sum4/1  "vd(t)"
  Product6/1 -> Sum2/1
  Product5/1 -> Sum6/2  "Rf*io(t)"
  Product2/1 -> Sum5/1  "Pp*wm(t)*Lq*iq(t)"
  1/Lq/1 -> Integrator/1  "iq_punto(t)"
  Sum6/1 -> 1/Lls/1
  [wm] -> Product6/1, Gain/1  "wm(t)"
  Product1/1 -> Tm(t)/1, [Tm]  "Tm(t)"
  Input1/1 -> Mux1/2  "vb(t)"
  Gain2/1 -> Park Transform1/2  "Pp*tita_m(t)"
  Input2/1 -> Mux1/3  "vc(t)"
  Mux1/1 -> Park Transform1/1
  Input/1 -> Mux1/1  "va(t)"
  [tita_m] -> Gain2/1
  Park Transform1/1 -> Demux1/1
  [Rf] -> Product3/2
  [Rf] -> Product4/2
  [Rf] -> Product5/2
  Integrator1/1 -> Product3/1, KEeq; KTeq/1(id(t)), Vector Concatenate/2  "id(t)"
  KEeq; KTeq/2(KTeq(t)) -> Display1/1, KTeq(t)/1
  KEeq; KTeq/1(KEeq(t)) -> KEeq(t)/1, Display/1
  [varKEeq] -> Product6/2
  Gain/1 -> Product2/1
  [varKTeq] -> Product1/1

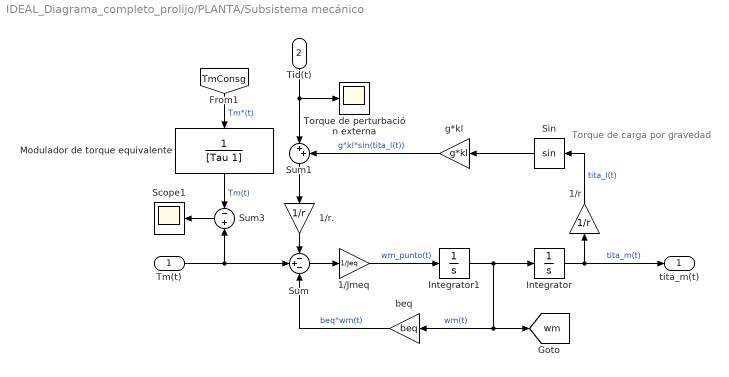
== system IDEAL_Diagrama_completo_prolijo/PLANTA/Subsistema mecánico ==
  note: Torque de carga por gravedad
  Tm(t) : Inport
  Tid(t) : Inport  Port=2
  1/Jmeq : Gain  Gain=1/Jeq
  1/r : Gain  Gain=1/r
  1/r. : Gain  Gain=1/r
  Integrator : Integrator  InitialCondition=tita0
  Integrator1 : Integrator  InitialCondition=wm0
  Modulador de torque equivalente : TransferFcn  Denominator=[Tau 1]
  Scope1 : Scope
  Sin : Trigonometry
  Sum : Sum  Inputs=-+-
  Sum1 : Sum  Inputs=|++
  Sum3 : Sum  Inputs=-|+
  Torque de perturbación externa : Scope
  beq : Gain  Gain=beq
  g*kl : Gain  Gain=g*kl
  tita_m(t) : Outport
  tag scope: wm=global
  wires:
  Integrator/1 -> tita_m(t)/1, 1/r/1  "tita_m(t)"
  1/r./1 -> Sum/1
  Integrator1/1 -> beq/1, [wm], Integrator/1  "wm(t)"
  1/r/1 -> Sin/1  "tita_l(t)"
  Sin/1 -> g*kl/1
  Sum/1 -> 1/Jmeq/1
  1/Jmeq/1 -> Integrator1/1  "wm_punto(t)"
  beq/1 -> Sum/3  "beq*wm(t)"
  Tid(t)/1 -> Sum1/1, Torque de perturbación externa/1
  Sum1/1 -> 1/r./1
  g*kl/1 -> Sum1/2  "g*kl*sin(tita_l(t))"
  [TmConsg] -> Modulador de torque equivalente/1  "Tm*(t)"
  Sum3/1 -> Scope1/1
  Modulador de torque equivalente/1 -> Sum3/1  "Tm(t)"
  Tm(t)/1 -> Sum/2, Sum3/2

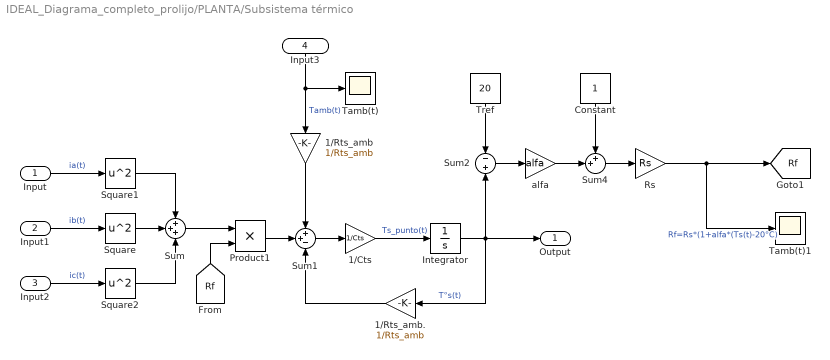
== system IDEAL_Diagrama_completo_prolijo/PLANTA/Subsistema térmico ==
  Input : Inport
  Input1 : Inport  Port=2
  Input2 : Inport  Port=3
  Input3 : Inport  Port=4
  1/Cts : Gain  Gain=1/Cts
  1/Rts_amb : Gain  Gain=1/Rts_amb
  1/Rts_amb. : Gain  Gain=1/Rts_amb
  Constant : Constant
  Integrator : Integrator  InitialCondition=Ts0
  Product1 : Product
  Rs : Gain  Gain=Rs
  Square : Math  Operator=square
  Square1 : Math  Operator=square
  Square2 : Math  Operator=square
  Sum : Sum  Inputs=+++
  Sum1 : Sum  Inputs=++-
  Sum2 : Sum  Inputs=-+
  Sum4 : Sum  Inputs=++|
  Tamb(t) : Scope
  Tamb(t)1 : Scope
  Tref : Constant  Value=20
  alfa : Gain  Gain=alfa
  Output : Outport
  tag scope: Rf=global
  wires:
  1/Rts_amb/1 -> Sum1/1
  Sum1/1 -> 1/Cts/1
  Product1/1 -> Sum1/2
  Sum/1 -> Product1/1
  Integrator/1 -> Sum2/2, Output/1, 1/Rts_amb./1  "T°s(t)"
  1/Cts/1 -> Integrator/1  "Ts_punto(t)"
  1/Rts_amb./1 -> Sum1/3
  Square/1 -> Sum/2
  Square1/1 -> Sum/1
  Square2/1 -> Sum/3
  Input/1 -> Square1/1  "ia(t)"
  Input1/1 -> Square/1  "ib(t)"
  Input2/1 -> Square2/1  "ic(t)"
  Sum2/1 -> alfa/1
  Constant/1 -> Sum4/1
  alfa/1 -> Sum4/2
  Rs/1 -> Tamb(t)1/1, [Rf]  "Rf=Rs*(1+alfa*(Ts(t)-20°C)"
  [Rf] -> Product1/2
  Tref/1 -> Sum2/1
  Sum4/1 -> Rs/1
  Input3/1 -> 1/Rts_amb/1, Tamb(t)/1  "Tamb(t)"

== system IDEAL_Diagrama_completo_prolijo/Subsystem/Espectro F ==
  abc : Inport  PortDimensions=3  SampleTime=Ts
  Model : Subsystem  AncestorBlock=|  DialogController=POWERSYS.PowerSysDialog
      | sps_lib/Control/PLL
      | (3ph)/Model
      settings: LibrarySourceBlock=|
      | sps_lib/Control/PLL
      | (3ph)/Model
  Freq : Outport  SampleTime=Ts  VectorParamsAs1DForOutWhenUnconnected=off
  wires:
  Model/1(Freq) -> Freq/1
  abc/1 -> Model/1(Vabc)

== system IDEAL_Diagrama_completo_prolijo/CONTROLADOR/PID/PID continuo (IDEAL) ==
  e_wm(t) : Inport
  Función de transferencia PID continuo equivalente : TransferFcn  Numerator=[ba Ksa Ksia]  Denominator=[1 0 0]
  Tm*´(t) : Outport
  wires:
  e_wm(t)/1 -> Función de transferencia PID continuo equivalente/1  "e_wm(t)"
  Función de transferencia PID continuo equivalente/1 -> Tm*´(t)/1  "Tm*´(t)"

== system IDEAL_Diagrama_completo_prolijo/CONTROLADOR/PID/PID discreto (REAL) ==
  note: Fixed-step-size = Ts
  e_wm(t) : Inport
  Función de transferencia PID discreto equivalente : DiscreteTransferFcn  Numerator=[0.1114 -0.2918 0.2552 -0.07479]  Denominator=[1 -3 3 -1]
  ZOH : ZeroOrderHold  SampleTime=Ts
  Tm*´(t) : Outport
  wires:
  e_wm(t)/1 -> ZOH/1  "e_wm(t)"
  ZOH/1 -> Función de transferencia PID discreto equivalente/1
  Función de transferencia PID discreto equivalente/1 -> Tm*´(t)/1  "Tm*´(t)"

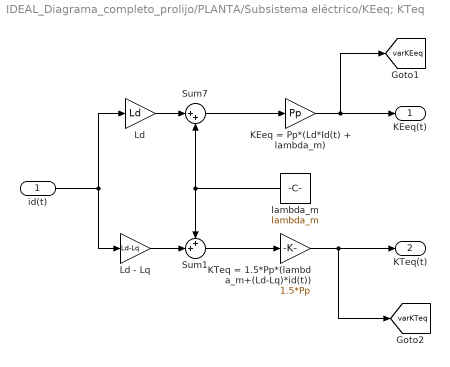
== system IDEAL_Diagrama_completo_prolijo/PLANTA/Subsistema eléctrico/KEeq; KTeq ==
  id(t) : Inport
  "KEeq = Pp*(Ld*Id(t) + lambda_m) " : Gain  Gain=Pp
  "KTeq = 1.5*Pp*(lambda_m+(Ld-Lq)*id(t)) " : Gain  Gain=1.5*Pp
  Ld : Gain  Gain=Ld
  Ld - Lq : Gain  Gain=Ld-Lq
  Sum1 : Sum  Inputs=++|
  Sum7 : Sum  Inputs=|++
  lambda_m : Constant  Value=lambda_m
  KEeq(t) : Outport
  KTeq(t) : Outport  Port=2
  tag scope: varKEeq=global, varKTeq=global
  wires:
  Ld/1 -> Sum7/1
  Sum7/1 -> "KEeq = Pp*(Ld*Id(t) + lambda_m) "/1
  "KTeq = 1.5*Pp*(lambda_m+(Ld-Lq)*id(t)) "/1 -> KTeq(t)/1, [varKTeq]
  Sum1/1 -> "KTeq = 1.5*Pp*(lambda_m+(Ld-Lq)*id(t)) "/1
  id(t)/1 -> Ld/1, Ld - Lq/1
  Ld - Lq/1 -> Sum1/2
  lambda_m/1 -> Sum1/1, Sum7/2
  "KEeq = Pp*(Ld*Id(t) + lambda_m) "/1 -> [varKEeq], KEeq(t)/1

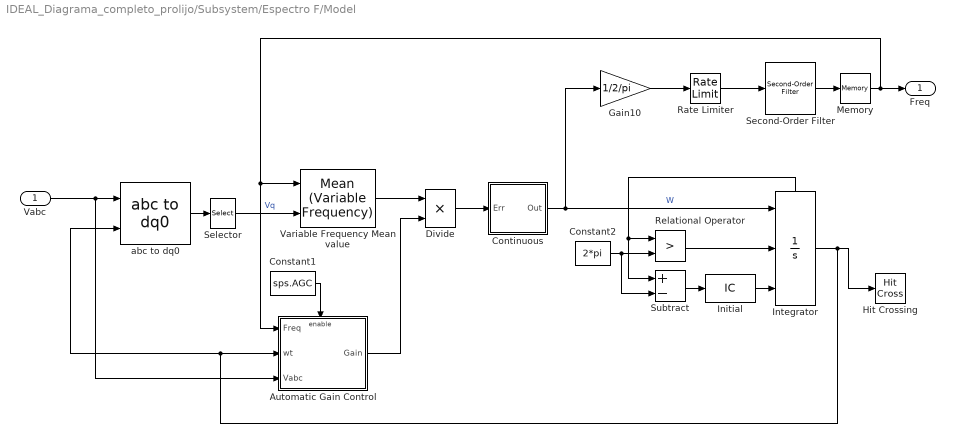
== system IDEAL_Diagrama_completo_prolijo/Subsystem/Espectro F/Model ==
  Vabc : Inport  PortDimensions=3
  Automatic Gain Control : Subsystem  TreatAsAtomicUnit=on
  Constant1 : Constant  Value=sps.AGC
  Constant2 : Constant  Value=2*pi
  Continuous : Subsystem  DialogController=POWERSYS.PowerSysDialog  VariantControl=PID_Continuous  mask(Continuous PID Controller){Kp=sps.Kp, Ki=sps.Ki, Kd=sps.Kd, TcD=sps.TcD, Par_Limits=[  inf 0 ], Init=2*pi*sps.Finit}
      mask prompts: Kp "Proportional gain (Kp):"; Ki "Integral gain (Ki):"; Kd "Derivative gain (Kd):"; TcD "Time constant for derivative filter (s):"; Par_Limits "Output limits: [ Upper   Lower ]"; Init "Output initial value:"
      mask help: This block implements a continuous PID controller.
      mask Display: disp('PID');
  Divide : Product
  Gain10 : Gain  Gain=1/2/pi  SaturateOnIntegerOverflow=on  OutDataTypeStr=Inherit: Same as input  ParamDataTypeStr=Inherit: Same as input
  Hit Crossing : HitCross  HitCrossingOffset=pi  HitCrossingDirection=falling  ShowOutputPort=off
  Initial : InitialCondition  Value=sps.Phase_Init*pi/180
  Integrator : Integrator  ExternalReset=rising  InitialConditionSource=external  InitialCondition=sps.Phase_Init*pi/180  LimitOutput=on  ShowStatePort=on
  Memory : Memory  InitialCondition=sps.Finit
  Rate Limiter : RateLimiter  RisingSlewLimit=sps.MaxRateChangeFreq  FallingSlewLimit=-sps.MaxRateChangeFreq
  Relational Operator : RelationalOperator  Operator=>  OutDataTypeStr=boolean  InputSameDT=off
  Second-Order Filter : spsSecondOrderFilterLib/Second-Order Filter  FilterType=Lowpass  Fo=sps.FilterCutOffFreq  Zeta=0.707  Ts=0  Initialize=on  Vac_Init=[0 0 sps.Finit]  Vdc_Init=sps.Finit  PlotResponse=off  FreqRange=[1 500 1]
      settings: LibrarySourceBlock=|
      | sps_lib/Control/Filters/Second-Order
      | Filter
  Selector : Selector  InputPortWidth=3  IndexOptions=Index vector (dialog)  Indices=2  OutputSizes=1
  Subtract : Sum  Inputs=+-
  Variable Frequency Mean value : spsMeanVariableFrequencyLib/Mean (Variable Frequency)  Finit=sps.Finit  Fmin=sps.Fmin  Vinit=0  Ts=0
      settings: LibrarySourceBlock=|
      | sps_lib/Sensors and Measurements/Mean
      | (Variable Frequency)
  abc to dq0 : spsabctodq0Lib/abc to dq0  Alignment=90 degrees behind phase A axis
  Freq : Outport  VectorParamsAs1DForOutWhenUnconnected=off
  wires:
  Continuous/1(Out) -> Gain10/1, Integrator/1  "W"
  Memory/1 -> Freq/1, Automatic Gain Control/1(Freq), Variable Frequency Mean value/1
  Constant1/1 -> Automatic Gain Control/Enable
  Divide/1 -> Continuous/1(Err)
  Automatic Gain Control/1(Gain) -> Divide/2
  Variable Frequency Mean value/1 -> Divide/1
  Vabc/1 -> abc to dq0/1, Automatic Gain Control/3(Vabc)
  abc to dq0/1 -> Selector/1
  Integrator/1 -> abc to dq0/2, Automatic Gain Control/2(wt), Hit Crossing/1
  Gain10/1 -> Rate Limiter/1
  Rate Limiter/1 -> Second-Order Filter/1
  Second-Order Filter/1 -> Memory/1
  Selector/1 -> Variable Frequency Mean value/2  "Vq"
  Constant2/1 -> Subtract/2, Relational Operator/2
  Relational Operator/1 -> Integrator/2
  Integrator/State -> Subtract/1, Relational Operator/1
  Subtract/1 -> Initial/1
  Initial/1 -> Integrator/3

== system IDEAL_Diagrama_completo_prolijo/Subsystem/Espectro F/Model/Automatic Gain Control ==
  Freq : Inport
  wt : Inport  Port=2
  Vabc : Inport  Port=3
  Enable : EnablePort  PropagateVarSize=During execution
  Math Function : Math  Operator=reciprocal  SignedPower=on
  Positive-Sequence (PLL-Driven) : spsPositiveSequencePLLDrivenLib/Positive-Sequence (PLL-Driven)  Finit=sps.Finit  Fmin=sps.Fmin  InInit=[1 0]  Ts=0
      settings: LibrarySourceBlock=|
      | sps_lib/Sensors and Measurements/Positive-Sequence
      | (PLL-Driven)
  Saturation : Saturate  UpperLimit=inf  LowerLimit=eps
  Terminator1 : Terminator
  Gain : Outport  InitialOutput=[1]  VectorParamsAs1DForOutWhenUnconnected=off
  wires:
  Saturation/1 -> Math Function/1
  Freq/1 -> Positive-Sequence (PLL-Driven)/1
  Vabc/1 -> Positive-Sequence (PLL-Driven)/3
  Math Function/1 -> Gain/1
  wt/1 -> Positive-Sequence (PLL-Driven)/2
  Positive-Sequence (PLL-Driven)/2 -> Terminator1/1
  Positive-Sequence (PLL-Driven)/1 -> Saturation/1

== system IDEAL_Diagrama_completo_prolijo/Subsystem/Espectro F/Model/Continuous ==
  Err : Inport  SampleTime=0
  Integrator : Integrator  InitialCondition=Init  LimitOutput=on  UpperSaturationLimit=Par_Limits(1)  LowerSaturationLimit=Par_Limits(2)
  Kp4 : Gain  Gain=Kp  SaturateOnIntegerOverflow=on  SampleTime=0  OutDataTypeStr=Inherit: Same as input  ParamDataTypeStr=Inherit: Same as input
  Kp5 : Gain  Gain=Ki  SaturateOnIntegerOverflow=on  SampleTime=0  OutDataTypeStr=Inherit: Same as input  ParamDataTypeStr=Inherit: Same as input
  Kp6 : Gain  Gain=Kd  SaturateOnIntegerOverflow=on  SampleTime=0  OutDataTypeStr=Inherit: Same as input  ParamDataTypeStr=Inherit: Same as input
  Saturation2 : Saturate  UpperLimit=Par_Limits(1)  LowerLimit=Par_Limits(2)  SampleTime=0
  Sum6 : Sum  Inputs=+++  InputSameDT=on  SaturateOnIntegerOverflow=on  SampleTime=0  OutDataTypeStr=Inherit: Same as first input
  Transfer Fcn : TransferFcn  Numerator=[1 0]  Denominator=[TcD 1]
  Out : Outport  SampleTime=0  InitialOutput=0  VectorParamsAs1DForOutWhenUnconnected=off
  wires:
  Saturation2/1 -> Out/1
  Err/1 -> Kp4/1, Kp5/1, Kp6/1
  Sum6/1 -> Saturation2/1
  Kp5/1 -> Integrator/1
  Kp6/1 -> Transfer Fcn/1
  Kp4/1 -> Sum6/1
  Integrator/1 -> Sum6/2
  Transfer Fcn/1 -> Sum6/3
